simulink model "hyun_Wiper_System"  (R2022b)
settings: Solver=FixedStepAuto  StartTime=0.0  StopTime=inf  FixedStep=0.001  RelTol=1e-3
libraries: arduinolib x4, dspswit3 x1
settings Model: ExtModeTrigDuration=2  Creator=현대오토1  LastModifiedBy=현대오토18
settings OptimizationCC: EnhancedBackFolding=on  PassReuseOutputArgsAs=Individual arguments  ZeroExternalMemoryAtStartup=off  ZeroInternalMemoryAtStartup=off  MaxStackSize=64  OptimizeBlockOrder=speed  DifferentSizesBufferReuse=on  OptimizationCustomize=off  EfficientTunableParamExpr=on
settings DebuggingCC: MultiTaskRateTransMsg=warning  ParameterTunabilityLossMsg=error
settings HardwareCC: ProdBitPerInt=16  ProdBitPerPointer=16  ProdBitPerSizeT=16  ProdBitPerPtrDiffT=16  ProdLargestAtomicFloat=None  ProdWordSize=8  ProdHWDeviceType=Atmel->AVR
settings SFSimCC: MATLABDynamicMemAlloc=off
settings RTWCC: Description=Embedded Coder  SystemTargetFile=ert.tlc  HardwareBoard=Arduino Mega 2560  TLCOptions=-aInlineSetEventsForThisBaseRateFcn=TLC_FALSE -aSuppressMultiTaskScheduler=TLC_FALSE -aRateBasedStepFcn=1  TemplateMakefile=ert_default_tmf  Toolchain=Arduino AVR  BuildConfiguration=Faster Runs
settings CodeAppCC: ForceParamTrailComments=on  IgnoreCustomStorageClasses=off  OperatorAnnotations=on  SimulinkDataObjDesc=on  SFDataObjDesc=on  InsertBlockDesc=on
settings ERTTargetCC: SupportContinuousTime=on  SupportVariableSizeSignals=on  ExtModeTransport=3  ExtModeStaticAlloc=on  ExtModeAutomaticAllocSize=off  ExtModeStaticAllocSize=2048  ExtModeMexFile=ext_xcp  ExtModeIntrfLevel=Level2 - Open

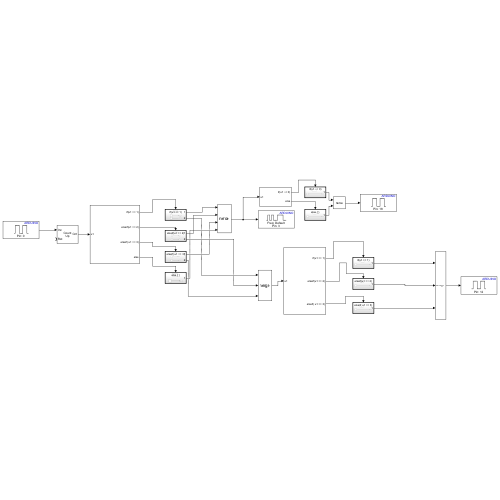
[thumbnail: Simulink's stored preview of the top-level diagram]
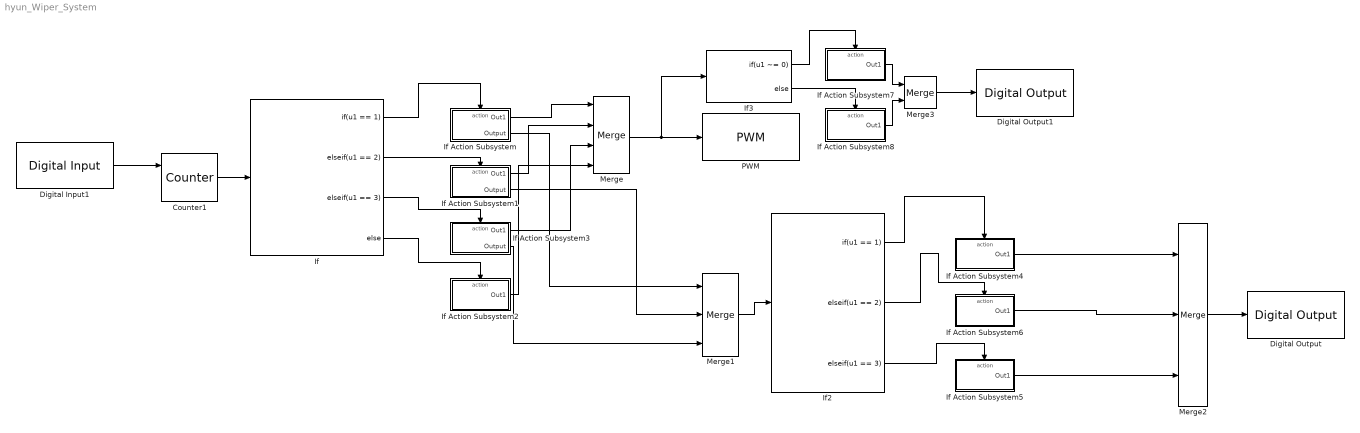
== system hyun_Wiper_System ==
  Counter1 : dspswit3/Counter  Direction=Up  CountEvent=Falling edge  CounterSize=User defined  MaxCount=3  InitialCount=0  Output=Count  HitValue=32  ResetInput=on  SamplesPerFrame=1  Ts=1  CntDtype=int8  HitDtype=Logical
  Digital Input1 : arduinolib/Digital Input  pinNumber=0  mode=Default  Direction=input  SampleTime=0.01  blockPlatform=arduino
  Digital Output : arduinolib/Digital Output  pinNumber=12  Direction=output  blockPlatform=arduino
  Digital Output1 : arduinolib/Digital Output  pinNumber=18  Direction=output  blockPlatform=arduino
  If : If  IfExpression=u1 == 1  ElseIfExpressions=u1 == 2, u1 == 3
  If Action Subsystem : Subsystem  TreatAsAtomicUnit=on
  If Action Subsystem1 : Subsystem  TreatAsAtomicUnit=on
  If Action Subsystem2 : Subsystem  TreatAsAtomicUnit=on
  If Action Subsystem3 : Subsystem  TreatAsAtomicUnit=on
  If Action Subsystem4 : Subsystem  TreatAsAtomicUnit=on
  If Action Subsystem5 : Subsystem  TreatAsAtomicUnit=on
  If Action Subsystem6 : Subsystem  TreatAsAtomicUnit=on
  If Action Subsystem7 : Subsystem  TreatAsAtomicUnit=on
  If Action Subsystem8 : Subsystem  TreatAsAtomicUnit=on
  If2 : If  IfExpression=u1 == 1  ElseIfExpressions=u1 == 2, u1 == 3  ShowElse=off
  If3 : If  IfExpression=u1 ~= 0
  Merge : Merge  Inputs=4
  Merge1 : Merge  Inputs=3
  Merge2 : Merge  Inputs=3
  Merge3 : Merge
  PWM : arduinolib/PWM  pinNumber=3  frequencyType=Default  desiredFrequency=490.2  achievableFrequency=490.2
  wires:
  Digital Input1/1 -> Counter1/1
  Counter1/1 -> If/1
  If/1 -> If Action Subsystem/Action
  If/2 -> If Action Subsystem1/Action
  If/3 -> If Action Subsystem3/Action
  If/4 -> If Action Subsystem2/Action
  If Action Subsystem/1(Out1) -> Merge/1
  If Action Subsystem1/1(Out1) -> Merge/2
  If Action Subsystem3/1(Out1) -> Merge/3
  If Action Subsystem2/1(Out1) -> Merge/4
  Merge/1 -> If3/1, PWM/1
  If Action Subsystem/2(Output) -> Merge1/1
  If Action Subsystem1/2(Output) -> Merge1/2
  If Action Subsystem3/2(Output) -> Merge1/3
  Merge1/1 -> If2/1
  If2/1 -> If Action Subsystem4/Action
  If2/2 -> If Action Subsystem6/Action
  If2/3 -> If Action Subsystem5/Action
  If Action Subsystem4/1(Out1) -> Merge2/1
  If Action Subsystem6/1(Out1) -> Merge2/2
  If Action Subsystem5/1(Out1) -> Merge2/3
  Merge2/1 -> Digital Output/1
  If3/1 -> If Action Subsystem7/Action
  If3/2 -> If Action Subsystem8/Action
  If Action Subsystem7/1(Out1) -> Merge3/1
  If Action Subsystem8/1(Out1) -> Merge3/2
  Merge3/1 -> Digital Output1/1

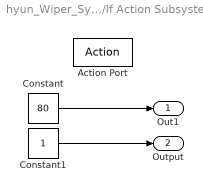
== system hyun_Wiper_System/If Action Subsystem ==
  Action Port : ActionPort  ActionPortLabel=if(u1 == 1)
  Constant : Constant  Value=80
  Constant1 : Constant
  Out1 : Outport
  Output : Outport  Port=2
  wires:
  Constant/1 -> Out1/1
  Constant1/1 -> Output/1

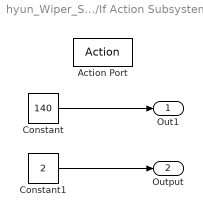
== system hyun_Wiper_System/If Action Subsystem1 ==
  Action Port : ActionPort  ActionPortLabel=elseif(u1 == 2)
  Constant : Constant  Value=140
  Constant1 : Constant  Value=2
  Out1 : Outport
  Output : Outport  Port=2
  wires:
  Constant/1 -> Out1/1
  Constant1/1 -> Output/1

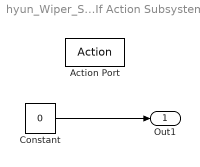
== system hyun_Wiper_System/If Action Subsystem2 ==
  Action Port : ActionPort  ActionPortLabel=else
  Constant : Constant  Value=0
  Out1 : Outport
  wires:
  Constant/1 -> Out1/1

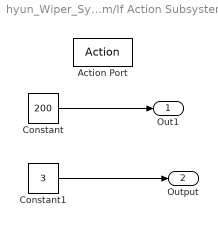
== system hyun_Wiper_System/If Action Subsystem3 ==
  Action Port : ActionPort  ActionPortLabel=elseif( u1 == 3)
  Constant : Constant  Value=200
  Constant1 : Constant  Value=3
  Out1 : Outport
  Output : Outport  Port=2
  wires:
  Constant/1 -> Out1/1
  Constant1/1 -> Output/1

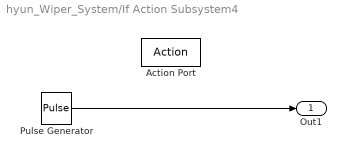
== system hyun_Wiper_System/If Action Subsystem4 ==
  Action Port : ActionPort  ActionPortLabel=if(u1 == 1)
  Pulse Generator : DiscretePulseGenerator  PulseType=Time based  PulseWidth=50
  Out1 : Outport
  wires:
  Pulse Generator/1 -> Out1/1

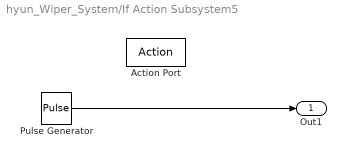
== system hyun_Wiper_System/If Action Subsystem5 ==
  Action Port : ActionPort  ActionPortLabel=elseif( u1 == 3)
  Pulse Generator : DiscretePulseGenerator  PulseType=Time based  Period=6  PulseWidth=50
  Out1 : Outport
  wires:
  Pulse Generator/1 -> Out1/1

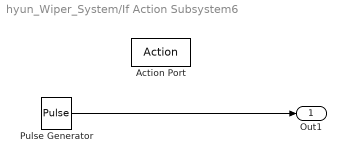
== system hyun_Wiper_System/If Action Subsystem6 ==
  Action Port : ActionPort  ActionPortLabel=elseif(u1 == 2)
  Pulse Generator : DiscretePulseGenerator  PulseType=Time based  Period=4  PulseWidth=50
  Out1 : Outport
  wires:
  Pulse Generator/1 -> Out1/1

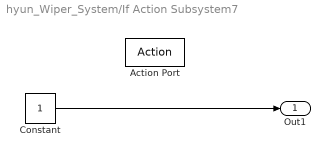
== system hyun_Wiper_System/If Action Subsystem7 ==
  Action Port : ActionPort  ActionPortLabel=if(u1 ~= 0)
  Constant : Constant
  Out1 : Outport
  wires:
  Constant/1 -> Out1/1

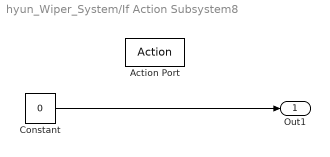
== system hyun_Wiper_System/If Action Subsystem8 ==
  Action Port : ActionPort  ActionPortLabel=else
  Constant : Constant  Value=0
  Out1 : Outport
  wires:
  Constant/1 -> Out1/1
